simulink model "example_LineFollower"  (Simulink 7.0)
settings: Solver=FixedStepDiscrete  StartTime=0.0  StopTime=inf  FixedStep=20  MaxStep=1  RelTol=1e-3
libraries: lib_robotinohardware x8, simulink x1
settings Model: Creator=indorewala  LastModifiedBy=indorewala
settings DebuggingCC: SaveWithParameterizedLinksMsg=none  SignalResolutionControl=TryResolveAllWithWarning  MultiTaskDSMMsg=warning  MultiTaskCondExecSysMsg=none
settings RTWCC: IncludeERTFirstTime=on
settings GRTTargetCC: TargetFcnLib=ansi_tfl_tmw.mat

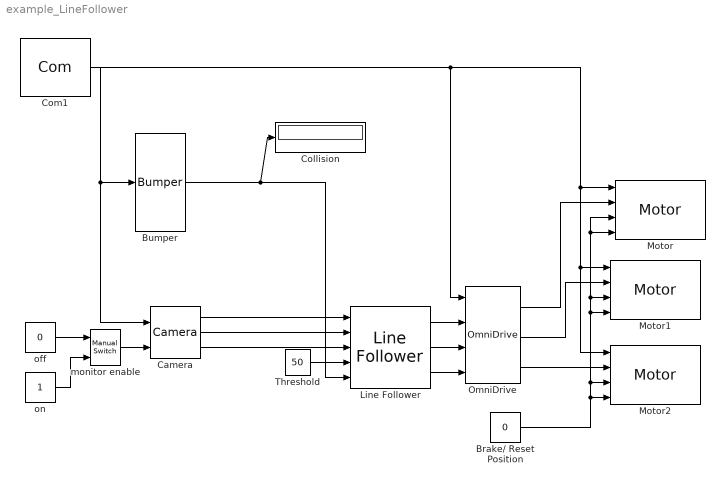
== system example_LineFollower ==
  Brake/ Reset Position : Constant  Value=0  OutDataType=sfix(16)  OutScaling=2^0
  Bumper : lib_robotinohardware/Bumper
  Camera : lib_robotinohardware/Camera
  Collision : Display
  Com1 : lib_robotinohardware/Com  ip='127.0.0.1'
  Line Follower : lib_robotinohardware/Line Follower
  Motor : lib_robotinohardware/Motor  num=0  kp=0.9  ki=0.1  kd=0
  Motor1 : lib_robotinohardware/Motor  num=1  kp=0.9  ki=0.1  kd=0
  Motor2 : lib_robotinohardware/Motor  num=2  kp=0.9  ki=0.1  kd=0
  OmniDrive : lib_robotinohardware/OmniDrive
  Threshold : Constant  Value=50  OutDataType=sfix(16)  OutScaling=2^0
  monitor enable : simulink/Signal Routing/Manual Switch  SystemSampleTime=-1  sw=0  action=0  varsize=off
  off : Constant  Value=0  OutDataType=sfix(16)  OutScaling=2^0
  on : Constant  OutDataType=sfix(16)  OutScaling=2^0
  wires:
  Com1/1 -> Bumper/1, Camera/1, Motor1/1, Motor2/1, Motor/1, OmniDrive/1
  Camera/1 -> Line Follower/1
  Camera/2 -> Line Follower/2
  Camera/3 -> Line Follower/3
  Bumper/1 -> Collision/1, Line Follower/5
  Threshold/1 -> Line Follower/4
  Line Follower/3 -> OmniDrive/4
  monitor enable/1 -> Camera/2
  off/1 -> monitor enable/1
  on/1 -> monitor enable/2
  Line Follower/1 -> OmniDrive/2
  Line Follower/2 -> OmniDrive/3
  OmniDrive/1 -> Motor/2
  OmniDrive/2 -> Motor1/2
  OmniDrive/3 -> Motor2/2
  Brake/ Reset Position/1 -> Motor/4, Motor/3, Motor1/3, Motor1/4, Motor2/3, Motor2/4
